simulink model "robot_ver_rotation"  (R2022b)
settings: Solver=VariableStepAuto  StartTime=0.0  StopTime=10.0  RelTol=1e-3
values from neighbouring files (symbols this model uses):
  r = 0.15    [robot_obstacle_parameters.m]
settings Model: Creator=rplatz  LastModifiedBy=rplatz
settings ModelReferenceCC: EnableRefExpFcnMdlSchedulingChecks=on

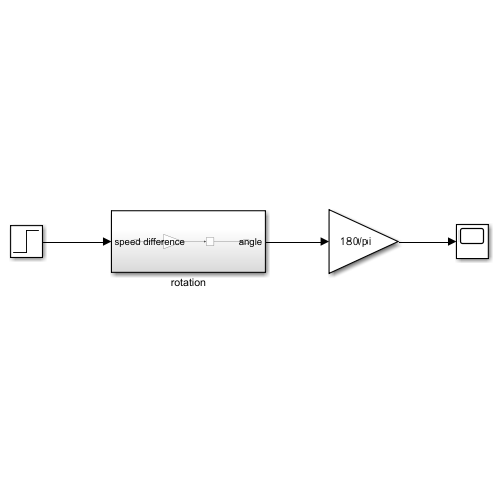
[thumbnail: Simulink's stored preview of the top-level diagram]
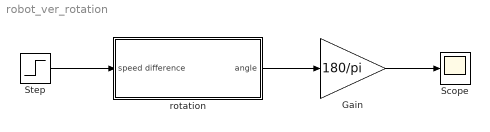
== system robot_ver_rotation ==
  Gain : Gain  Gain=180/pi
  Scope : Scope
  Step : Step  SampleTime=0
  rotation : Subsystem
  wires:
  Step/1 -> rotation/1(speed difference)
  rotation/1(angle) -> Gain/1
  Gain/1 -> Scope/1

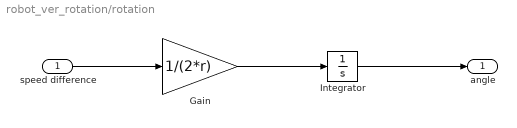
== system robot_ver_rotation/rotation ==
  speed difference : Inport
  Gain : Gain  Gain=1/(2*r)
  Integrator : Integrator
  angle : Outport
  wires:
  Gain/1 -> Integrator/1
  Integrator/1 -> angle/1
  speed difference/1 -> Gain/1
